simulink model "model"  (R2019a)
settings: Solver=VariableStepAuto  StartTime=0.0  StopTime=10.0  RelTol=1e-3
values from neighbouring files (symbols this model uses):
  a = 0    [model.m]    (also in model_config.m = 1)
  b = 0    [model.m]    (also in model_config.m = 1)
  c_f = 0    [model.m]    (also in model_config.m = 200)
  c_r = 0    [model.m]    (also in model_config.m = 200)
  g = 9.8    [model.m]    (also in model_config.m)
  h = 0    [model.m]    (also in model_config.m = 0.1)
  l = 0    [model.m]    (also in model_config.m = 2)
  m = 200    [model.m]    (also in model_config.m)
  mu = 0    [model.m]    (also in model_config.m = 1)
  P_f = 1    [model.m]    (also in model_config.m)
  P_r = P_f    (= 1)    [model.m]    (also in model_config.m)
  steering_angle = 0    [model.m]    (also in model_config.m = 1)
  vel_lat = 0    [model.m]    (also in model_config.m = 10)
  vel_lon = 0    [model.m]    (also in model_config.m = 10)
  W = 200    [model.m]    (also in model_config.m)
  yaw_angle = 0    [model.m]    (also in model_config.m = -5)
settings Model: Creator=jacoboffersen  LastModifiedBy=jacoboffersen

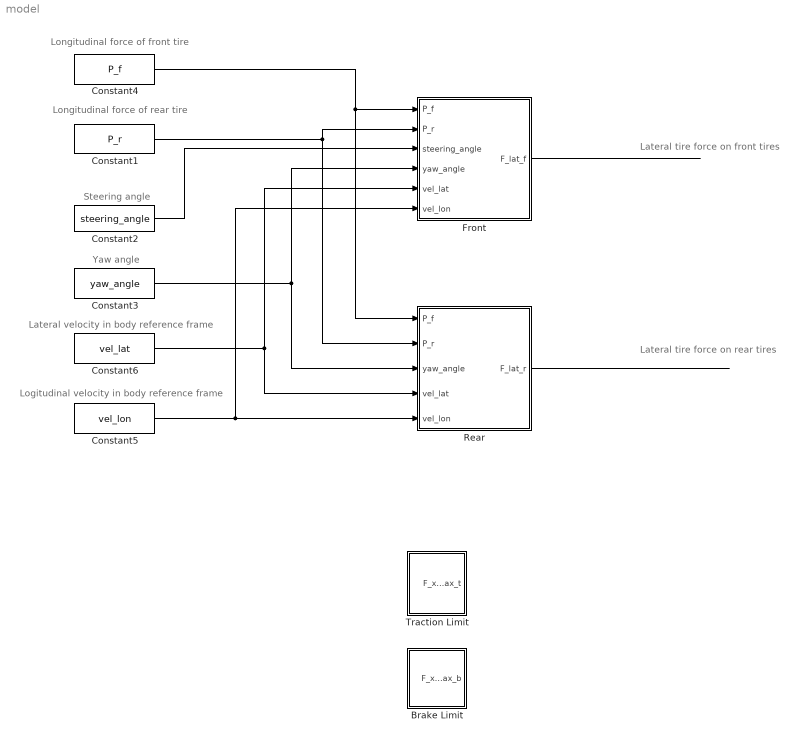
== system model ==
  note: Logitudinal velocity in body reference frame
  note: Yaw angle
  note: Steering angle
  note: Longitudinal force of rear tire
  note: Longitudinal force of front tire
  note: Lateral tire force on rear tires
  note: Lateral velocity in body reference frame
  note: Lateral tire force on front tires
  "Brake Limit " : Subsystem
  Constant1 : Constant  Value=P_r
  Constant2 : Constant  Value=steering_angle
  Constant3 : Constant  Value=yaw_angle
  Constant4 : Constant  Value=P_f
  Constant5 : Constant  Value=vel_lon
  Constant6 : Constant  Value=vel_lat
  Front : Subsystem
  Rear : Subsystem
  "Traction Limit " : Subsystem
  wires:
  Front/1(F_lat_f) -> ?
  Rear/1(F_lat_r) -> ?
  Constant4/1 -> Rear/1(P_f), Front/1(P_f)
  Constant1/1 -> Rear/2(P_r), Front/2(P_r)
  Constant2/1 -> Front/3(steering_angle)
  Constant3/1 -> Rear/3(yaw_angle), Front/4(yaw_angle)
  Constant6/1 -> Rear/4(vel_lat), Front/5(vel_lat)
  Constant5/1 -> Front/6(vel_lon), Rear/5(vel_lon)

== system model/Brake Limit  ==
  Constant : Constant  Value=mu*(W/l)*(a+mu*h)
  F_x_max_b : Outport
  wires:
  Constant/1 -> F_x_max_b/1

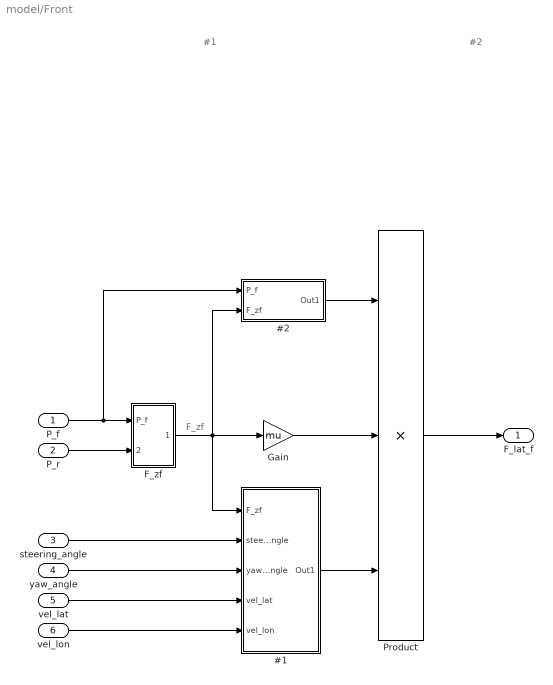
== system model/Front ==
  note: F_zf
  note: #1
  note: #2
  P_f : Inport
  P_r : Inport  Port=2
  steering_angle : Inport  Port=3
  yaw_angle : Inport  Port=4
  vel_lat : Inport  Port=5
  vel_lon : Inport  Port=6
  #1 : Subsystem
  #2 : Subsystem
  F_zf : Subsystem
  Gain : Gain  Gain=mu
  Product : Product  Inputs=3
  F_lat_f : Outport
  wires:
  #1/1(Out1) -> Product/3
  yaw_angle/1 -> #1/3(yaw_angle)
  vel_lat/1 -> #1/4(vel_lat)
  P_f/1 -> #2/1(P_f), F_zf/1(P_f)
  steering_angle/1 -> #1/2(steering_angle)
  F_zf/1(F_zf) -> #2/2(F_zf), #1/1(F_zf), Gain/1
  Gain/1 -> Product/2
  Product/1 -> F_lat_f/1
  P_r/1 -> F_zf/2(P_r)
  #2/1(Out1) -> Product/1
  vel_lon/1 -> #1/5(vel_lon)

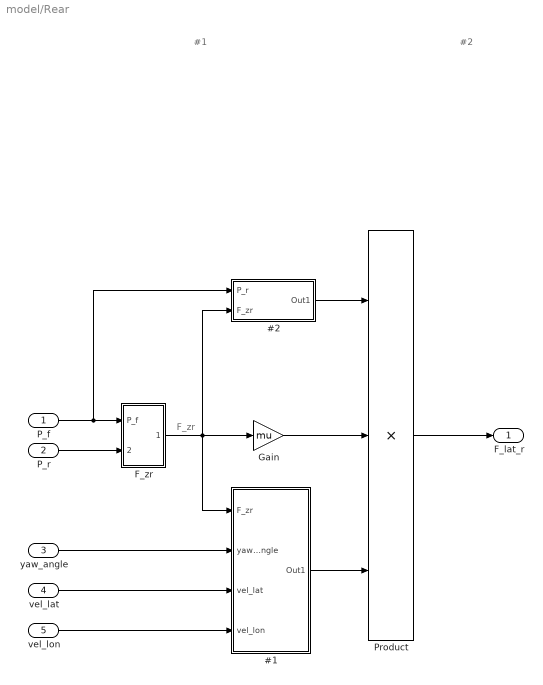
== system model/Rear ==
  note: F_zr
  note: #1
  note: #2
  P_f : Inport
  P_r : Inport  Port=2
  yaw_angle : Inport  Port=3
  vel_lat : Inport  Port=4
  vel_lon : Inport  Port=5
  #1 : Subsystem
  #2 : Subsystem
  F_zr : Subsystem
  Gain : Gain  Gain=mu
  Product : Product  Inputs=3
  F_lat_r : Outport
  wires:
  #1/1(Out1) -> Product/3
  yaw_angle/1 -> #1/2(yaw_angle)
  vel_lat/1 -> #1/3(vel_lat)
  P_f/1 -> #2/1(P_r), F_zr/1(P_f)
  F_zr/1(F_zr) -> #2/2(F_zr), #1/1(F_zr), Gain/1
  Gain/1 -> Product/2
  Product/1 -> F_lat_r/1
  P_r/1 -> F_zr/2(P_r)
  #2/1(Out1) -> Product/1
  vel_lon/1 -> #1/4(vel_lon)

== system model/Traction Limit  ==
  Constant5 : Constant  Value=(mu*(W*b)/l)/(1+mu*(h/l))
  F_x_max_t : Outport
  wires:
  Constant5/1 -> F_x_max_t/1

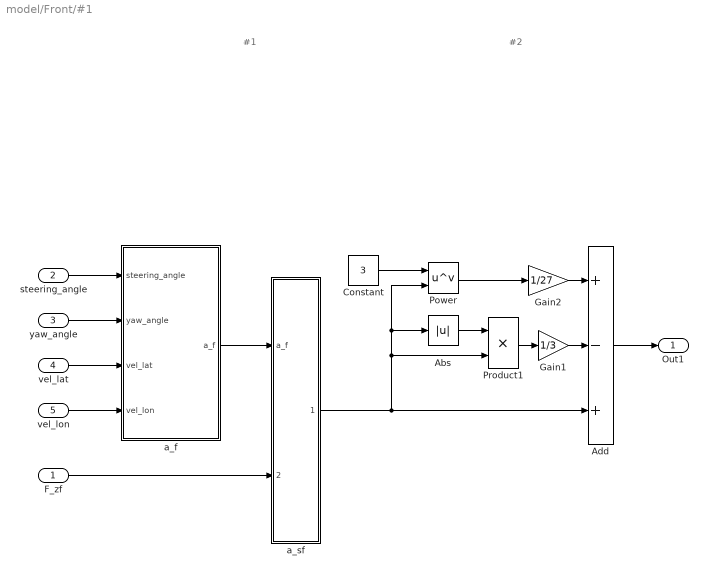
== system model/Front/#1 ==
  note: #1
  note: #2
  F_zf : Inport
  steering_angle : Inport  Port=2
  yaw_angle : Inport  Port=3
  vel_lat : Inport  Port=4
  vel_lon : Inport  Port=5
  Abs : Abs
  Add : Sum  Inputs=+-+
  Constant : Constant  Value=3
  Gain1 : Gain  Gain=1/3
  Gain2 : Gain  Gain=1/27
  Power : Math  Operator=pow  SaturateOnIntegerOverflow=on
  Product1 : Product
  a_f : Subsystem
  a_sf : Subsystem
  Out1 : Outport
  wires:
  Product1/1 -> Gain1/1
  vel_lon/1 -> a_f/4(vel_lon)
  Power/1 -> Gain2/1
  a_f/1(a_f) -> a_sf/1(a_f)
  Add/1 -> Out1/1
  yaw_angle/1 -> a_f/2(yaw_angle)
  Gain2/1 -> Add/1
  steering_angle/1 -> a_f/1(steering_angle)
  vel_lat/1 -> a_f/3(vel_lat)
  F_zf/1 -> a_sf/2(F_zf)
  a_sf/1(a_sf) -> Abs/1, Power/2, Product1/2, Add/3
  Constant/1 -> Power/1
  Abs/1 -> Product1/1
  Gain1/1 -> Add/2

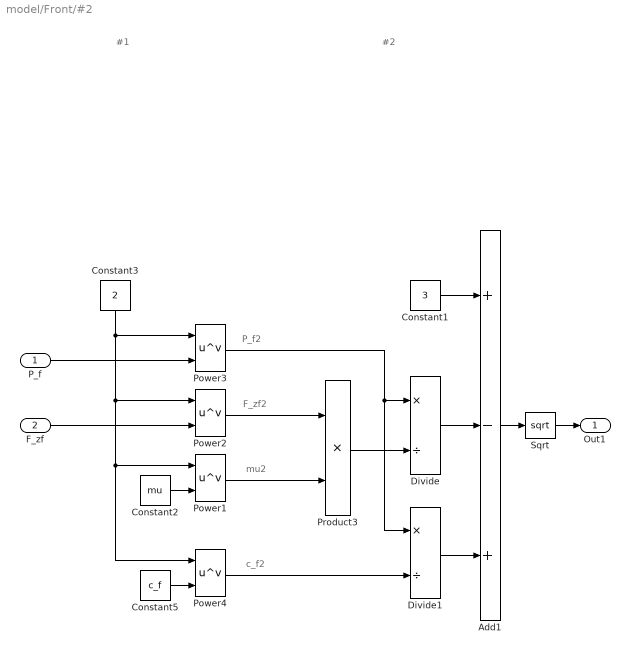
== system model/Front/#2 ==
  note: c_f2
  note: mu2
  note: F_zf2
  note: P_f2
  note: #1
  note: #2
  P_f : Inport
  F_zf : Inport  Port=2
  Add1 : Sum  Inputs=+-+
  Constant1 : Constant  Value=3
  Constant2 : Constant  Value=mu
  Constant3 : Constant  Value=2
  Constant5 : Constant  Value=c_f
  Divide : Product  Inputs=*/
  Divide1 : Product  Inputs=*/
  Power{1..4} (4 alike) : Math  Operator=pow  SaturateOnIntegerOverflow=on
  Product3 : Product
  Sqrt : Sqrt  SaturateOnIntegerOverflow=on
  Out1 : Outport
  wires:
  Power4/1 -> Divide1/2
  P_f/1 -> Power3/2
  Product3/1 -> Divide/2
  Constant1/1 -> Add1/1
  Divide1/1 -> Add1/3
  Power3/1 -> Divide1/1, Divide/1
  Divide/1 -> Add1/2
  Sqrt/1 -> Out1/1
  Add1/1 -> Sqrt/1
  Constant5/1 -> Power4/2
  Constant3/1 -> Power2/1, Power1/1, Power4/1, Power3/1
  Power1/1 -> Product3/2
  Constant2/1 -> Power1/2
  Power2/1 -> Product3/1
  F_zf/1 -> Power2/2

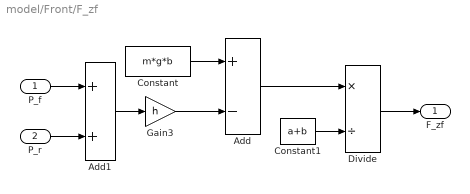
== system model/Front/F_zf ==
  P_f : Inport
  P_r : Inport  Port=2
  Add : Sum  Inputs=+-
  Add1 : Sum
  Constant : Constant  Value=m*g*b
  Constant1 : Constant  Value=a+b
  Divide : Product  Inputs=*/
  Gain3 : Gain  Gain=h
  F_zf : Outport
  wires:
  Add1/1 -> Gain3/1
  P_f/1 -> Add1/1
  P_r/1 -> Add1/2
  Constant/1 -> Add/1
  Gain3/1 -> Add/2
  Add/1 -> Divide/1
  Constant1/1 -> Divide/2
  Divide/1 -> F_zf/1

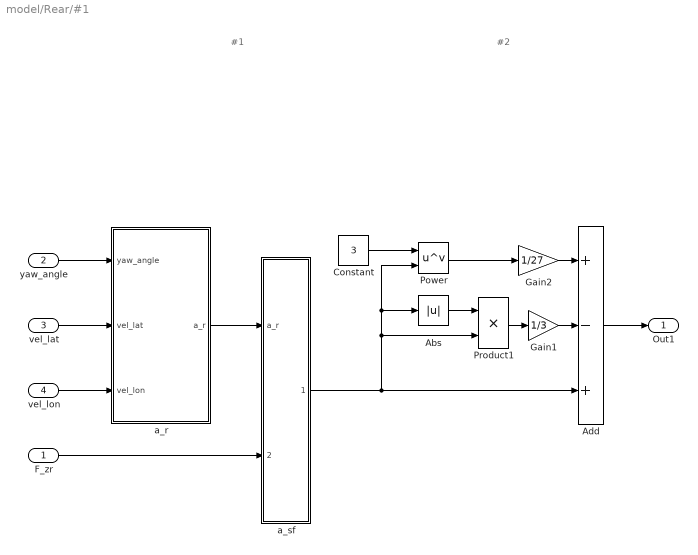
== system model/Rear/#1 ==
  note: #2
  note: #1
  F_zr : Inport
  yaw_angle : Inport  Port=2
  vel_lat : Inport  Port=3
  vel_lon : Inport  Port=4
  Abs : Abs
  Add : Sum  Inputs=+-+
  Constant : Constant  Value=3
  Gain1 : Gain  Gain=1/3
  Gain2 : Gain  Gain=1/27
  Power : Math  Operator=pow  SaturateOnIntegerOverflow=on
  Product1 : Product
  a_r : Subsystem
  a_sf : Subsystem
  Out1 : Outport
  wires:
  Product1/1 -> Gain1/1
  vel_lon/1 -> a_r/3(vel_lon)
  Power/1 -> Gain2/1
  a_r/1(a_r) -> a_sf/1(a_r)
  Add/1 -> Out1/1
  yaw_angle/1 -> a_r/1(yaw_angle)
  Gain2/1 -> Add/1
  vel_lat/1 -> a_r/2(vel_lat)
  F_zr/1 -> a_sf/2(F_zr)
  a_sf/1(a_sr) -> Abs/1, Power/2, Product1/2, Add/3
  Constant/1 -> Power/1
  Abs/1 -> Product1/1
  Gain1/1 -> Add/2

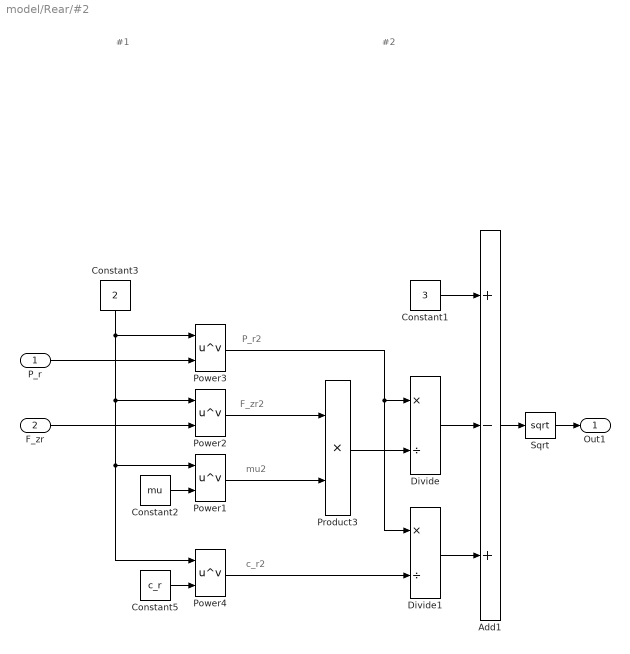
== system model/Rear/#2 ==
  note: c_r2
  note: mu2
  note: F_zr2
  note: P_r2
  note: #1
  note: #2
  P_r : Inport
  F_zr : Inport  Port=2
  Add1 : Sum  Inputs=+-+
  Constant1 : Constant  Value=3
  Constant2 : Constant  Value=mu
  Constant3 : Constant  Value=2
  Constant5 : Constant  Value=c_r
  Divide : Product  Inputs=*/
  Divide1 : Product  Inputs=*/
  Power{1..4} (4 alike) : Math  Operator=pow  SaturateOnIntegerOverflow=on
  Product3 : Product
  Sqrt : Sqrt  SaturateOnIntegerOverflow=on
  Out1 : Outport
  wires:
  Power4/1 -> Divide1/2
  P_r/1 -> Power3/2
  Product3/1 -> Divide/2
  Constant1/1 -> Add1/1
  Divide1/1 -> Add1/3
  Power3/1 -> Divide1/1, Divide/1
  Divide/1 -> Add1/2
  Sqrt/1 -> Out1/1
  Add1/1 -> Sqrt/1
  Constant5/1 -> Power4/2
  Constant3/1 -> Power2/1, Power1/1, Power4/1, Power3/1
  Power1/1 -> Product3/2
  Constant2/1 -> Power1/2
  Power2/1 -> Product3/1
  F_zr/1 -> Power2/2

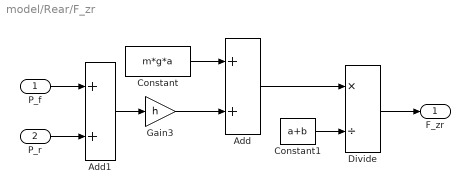
== system model/Rear/F_zr ==
  P_f : Inport
  P_r : Inport  Port=2
  Add : Sum
  Add1 : Sum
  Constant : Constant  Value=m*g*a
  Constant1 : Constant  Value=a+b
  Divide : Product  Inputs=*/
  Gain3 : Gain  Gain=h
  F_zr : Outport
  wires:
  Add1/1 -> Gain3/1
  P_f/1 -> Add1/1
  P_r/1 -> Add1/2
  Constant/1 -> Add/1
  Gain3/1 -> Add/2
  Add/1 -> Divide/1
  Constant1/1 -> Divide/2
  Divide/1 -> F_zr/1

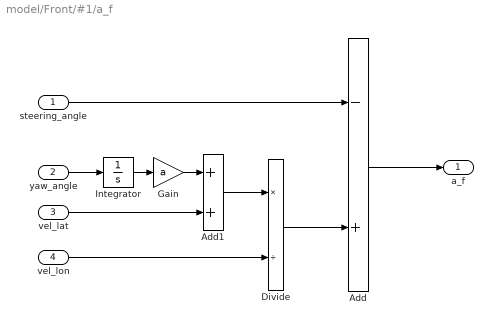
== system model/Front/#1/a_f ==
  steering_angle : Inport
  yaw_angle : Inport  Port=2
  vel_lat : Inport  Port=3
  vel_lon : Inport  Port=4
  Add : Sum  Inputs=-+
  Add1 : Sum
  Divide : Product  Inputs=*/
  Gain : Gain  Gain=a
  Integrator : Integrator
  a_f : Outport
  wires:
  Add/1 -> a_f/1
  steering_angle/1 -> Add/1
  yaw_angle/1 -> Integrator/1
  Integrator/1 -> Gain/1
  Gain/1 -> Add1/1
  vel_lat/1 -> Add1/2
  vel_lon/1 -> Divide/2
  Add1/1 -> Divide/1
  Divide/1 -> Add/2

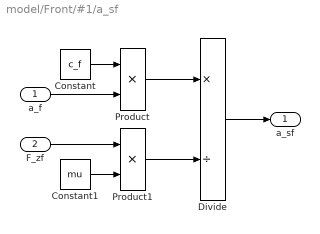
== system model/Front/#1/a_sf ==
  a_f : Inport
  F_zf : Inport  Port=2
  Constant : Constant  Value=c_f
  Constant1 : Constant  Value=mu
  Divide : Product  Inputs=*/
  Product : Product
  Product1 : Product
  a_sf : Outport
  wires:
  Divide/1 -> a_sf/1
  a_f/1 -> Product/2
  Constant/1 -> Product/1
  Constant1/1 -> Product1/2
  F_zf/1 -> Product1/1
  Product/1 -> Divide/1
  Product1/1 -> Divide/2

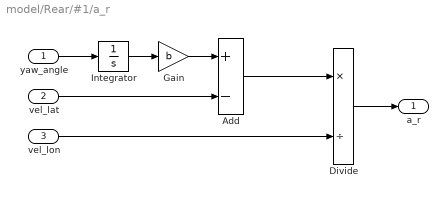
== system model/Rear/#1/a_r ==
  yaw_angle : Inport
  vel_lat : Inport  Port=2
  vel_lon : Inport  Port=3
  Add : Sum  Inputs=+-
  Divide : Product  Inputs=*/
  Gain : Gain  Gain=b
  Integrator : Integrator
  a_r : Outport
  wires:
  yaw_angle/1 -> Integrator/1
  Integrator/1 -> Gain/1
  Gain/1 -> Add/1
  Add/1 -> Divide/1
  Divide/1 -> a_r/1
  vel_lat/1 -> Add/2
  vel_lon/1 -> Divide/2

== system model/Rear/#1/a_sf ==
  a_r : Inport
  F_zr : Inport  Port=2
  Constant : Constant  Value=c_r
  Constant1 : Constant  Value=mu
  Divide : Product  Inputs=*/
  Product : Product
  Product1 : Product
  a_sr : Outport
  wires:
  Divide/1 -> a_sr/1
  a_r/1 -> Product/2
  Constant/1 -> Product/1
  Constant1/1 -> Product1/2
  F_zr/1 -> Product1/1
  Product/1 -> Divide/1
  Product1/1 -> Divide/2
